simulink model "Task7"  (R2023b)
settings: Solver=VariableStepAuto  StartTime=0.0  StopTime=1800  RelTol=1e-3
InitFcn:
  | run("Linear_Model.m")
values from neighbouring files (symbols this model uses):
  A_Lat = [Yv   Yp+w0   Yr-u0         gravity*cos(theta0)     0 ... (first row only)    [Linear_Model.m]
  A_Long = [Xu                    Xw                        -w0                            -gravity*cos(theta0) ... (first row only)    [Linear_Model.m]
  B_Lat = [Yda          Ydr ... (first row only)    [Linear_Model.m]
  B_Long = [Xde                         Xdth ... (first row only)    [Linear_Model.m]
  C_Lat = eye(5)    [Linear_Model.m]
  C_Long = eye(4)    [Linear_Model.m]
  D_Lat = zeros(5,2)    [Linear_Model.m]
  D_Long = zeros(4,2)    [Linear_Model.m]
  F_gravity_0 = mass*gravity*[sin(states_0(8)) ... (first row only)    [Data_edit.m]
  gravity = Airplane_data(52)    [Data_edit.m]
  Ixx = Airplane_data(53)    [Data_edit.m]
  Iyy = Airplane_data(54)    [Data_edit.m]
  Izz = Airplane_data(55)    [Data_edit.m]
  M0 = [0;0;0]    [Data_edit.m]
  mass = Airplane_data(51)    [Data_edit.m]
  Matrix_controls = [ 0             Xde             Xdth            0 ... (first row only)    [Data_edit.m]
  Matrix_states = [Xu   0   Xw  0   0   0   0 ... (first row only)    [Data_edit.m]
  p0 = states_0(4)    [Data_edit.m]
  phi0 = states_0(7)    [Data_edit.m]
  psi0 = states_0(9)    [Data_edit.m]
  q0 = states_0(5)    [Data_edit.m]
  r0 = states_0(6)    [Data_edit.m]
  states_0 = Airplane_data(4:15)    [Data_edit.m]
  theta0 = states_0(8)    [Data_edit.m]
  u0 = states_0(1)    [Data_edit.m]
  v0 = states_0(2)    [Data_edit.m]
  w0 = states_0(3)    [Data_edit.m]
undefined symbols (not defined in the file or in its folder): Earth, sigbuilder_block, WGS84
libraries: simulink_extras x35, cstblocks x17, slpidlib x12, aerolibasang x2, aerolibfltsims x2, shared6dof x1, dspsigops x1, aerolibtransform2 x1
(part 1 of 2)
settings Model: Creator=saifg  LastModifiedBy=saifg

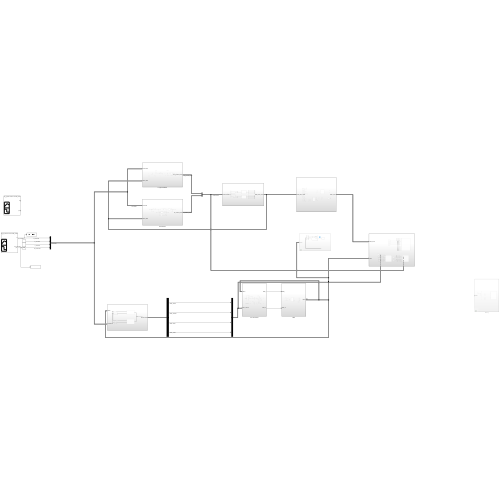
[thumbnail: Simulink's stored preview of the top-level diagram]
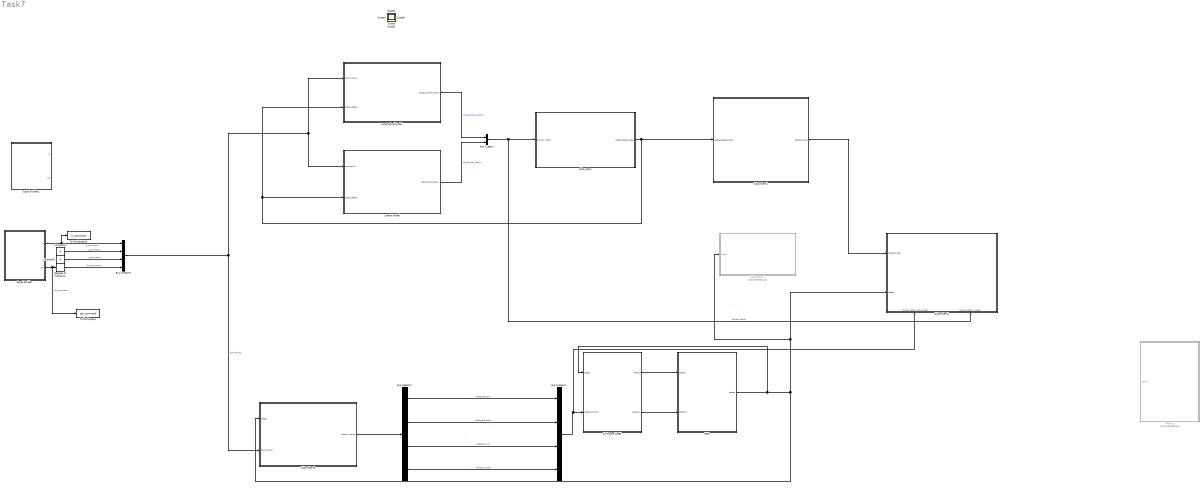
== system Task7 ==
  Air Frame Model : Subsystem
  Bus Creator : BusCreator  Inputs=2
  Bus Creator4 : BusCreator  Inputs=4
  Bus Creator5 : BusCreator  Inputs=4
  Bus Selector : BusSelector  OutputSignals=Lat_Control_Action.delta_aileron,Long_Control_Action.delta_elevator,Long_Control_Action.delta_thrust,Lat_Control_Action.delta_ruuder
  Constant4 : Constant  Value=0
  Constant5 : Constant  Value=0
  Degrees to Radians2 : simulink_extras/Transformations/Degrees to Radians
  "Lateral Model " : Subsystem
  Longitudinal Model : Subsystem
  Plotting : Subsystem  Commented=on
  RBD : Subsystem
  Signal Builder : Subsystem  Tag=STV Subsys  LoadFcn=sigbuilder_block('load');  StartFcn=sigbuilder_block('start');  StopFcn=sigbuilder_block('stop');  ClipboardFcn=sigbuilder_block('clipboard');  mask(Sigbuilder block){tuvar=[0:10]}
      mask help: Simulink:masks:SigbuilderBlock_MD
      mask init:
      | if ~strcmp(get_param(bdroot(gcbh),'SimulationStatus'),'stopped') tuvar = sigbuilder_block('maskInit'); end
      settings: CopyFcn=sigbuilder_block('copy');  DeleteFcn=sigbuilder_block('delete');  ModelCloseFcn=sigbuilder_block('modelClose');  PreSaveFcn=sigbuilder_block('preSave');  PauseFcn=sigbuilder_block('pause');  ContinueFcn=sigbuilder_block('continue');  NameChangeFcn=sigbuilder_block('namechange');  OpenFcn=sigbuilder_block('open',[5.4 36 1141.2 516.6 ]);  CloseFcn=sigbuilder_block('close');
      mask Display: plot(0, 0, 100, 100,[2, 2, 32, 32, 2], [68, 8, 8, 68, 68],[32, 2], [38, 38], [32, 19, 2],[53, 60, 44], [32, 17, 17, 2],[16, 16, 31, 31]);txt = getActiveGroup(gcbh);text(2, 100, txt,'verticalAlignment', 'top');
  Signal Builder1 : Subsystem  Tag=STV Subsys  LoadFcn=sigbuilder_block('load');  StartFcn=sigbuilder_block('start');  StopFcn=sigbuilder_block('stop');  ClipboardFcn=sigbuilder_block('clipboard');  mask(Sigbuilder block){tuvar=[0:10]}
      mask help: Simulink:masks:SigbuilderBlock_MD
      mask init:
      | if ~strcmp(get_param(bdroot(gcbh),'SimulationStatus'),'stopped') tuvar = sigbuilder_block('maskInit'); end
      settings: CopyFcn=sigbuilder_block('copy');  DeleteFcn=sigbuilder_block('delete');  ModelCloseFcn=sigbuilder_block('modelClose');  PreSaveFcn=sigbuilder_block('preSave');  PauseFcn=sigbuilder_block('pause');  ContinueFcn=sigbuilder_block('continue');  NameChangeFcn=sigbuilder_block('namechange');  OpenFcn=sigbuilder_block('open',[5.4 36 1141.2 516.6 ]);  CloseFcn=sigbuilder_block('close');
      mask Display: plot(0, 0, 100, 100,[2, 2, 32, 32, 2], [68, 8, 8, 68, 68],[32, 2], [38, 38], [32, 19, 2],[53, 60, 44], [32, 17, 17, 2],[16, 16, 31, 31]);txt = getActiveGroup(gcbh);text(2, 100, txt,'verticalAlignment', 'top');
  Subsystem : Subsystem
  Subsystem1 : Subsystem
  Subsystem2 : Subsystem
      settings: PortSchema="{\"entries\":[{\"content\":{\"sides\":[{\"content\":{\"connectorIds\":[\"In1\",\"In2\"]},\"type\":\"ConnectorPlacement.EquallySpacedRectSide\",\"uuid\":\"ba0f1933-2a67-495f-a755-837ae570be10\"},{\"content\":{\"side\":\"RIGHT\"},\"type\":\"ConnectorPlacement.EquallySpacedRectSide\",\"uuid\":\"3de798a5-8bce-4885-8633-4329ea784db0\"},{\"content\":{\"side\":\"TOP\"},\"type\":\"ConnectorPlacement.EquallySpacedRectSide\",\"uuid\":\"6ce253ea-975e-40d2-945b-e7cccea3a524\"},{\"content\":{\"connectorIds\":[\"In3\",\"In4\"],\"side\":\"BOTTOM\"},\"type\":\"ConnectorPlacement.EquallySpacedRectSide\",\"uuid\":\"4e7a2a38-3005-49de-8745-c2ef2fbabb58\"}]},\"type\":\"ConnectorPlacement.EquallySpacedConnector\",\"uuid\":\"bc25b1a9-6a92-4f96-820d-23b739a2dded\"}],\"packageUris\":[\"http://schema.mathworks.com/mf0/Connector/R2020b\"],\"version\":\"1.0\"}"
  Subsystem3 : Subsystem
  Subsystem4 : Subsystem  Commented=on
  To Workspace : ToWorkspace  VariableName=psi_command  SampleTime=-1
  To Workspace1 : ToWorkspace  VariableName=H_Command  SampleTime=-1
  Scope{,1..4} (5 alike) : Scope
  wires:
  "Lateral Model "/1(Lat_control_action) -> Bus Creator/2  "Lat_Control_Action"
  Longitudinal Model/1(Long_Control_action) -> Bus Creator/1  "Long_Control_Action"
  Bus Creator/1 -> Subsystem2/4(Conrol Action  Linear), Subsystem/1(Control Action)  "Control Action"
  Subsystem/1(delta_sates_Linear) -> Subsystem1/1(delta_sates_Linear), Longitudinal Model/2(delta_states), "Lateral Model "/2(delta_states)
  Bus Creator5/1 -> Subsystem3/2(Commands), Longitudinal Model/1(Commands), "Lateral Model "/1(command)  "Commands"
  Subsystem1/1(states_linear) -> Subsystem2/1(states_linear)
  Bus Creator4/1 -> Subsystem2/3(Conrol Action Non Linear), Air Frame Model/2(delta_controls)
  RBD/1(states) -> Air Frame Model/1(states), Subsystem4/1(States), Subsystem2/2(states), Subsystem3/1(states)
  Air Frame Model/2(delta_m) -> RBD/2(delta_M)
  Air Frame Model/1(delta_f) -> RBD/1(delta_f)
  Constant5/1 -> Bus Creator5/3  "r_command"
  Constant4/1 -> Bus Creator5/2  "u_command"
  Degrees to Radians2/1 -> Bus Creator5/4  "Psi_command"
  Subsystem3/1(Control Action) -> Bus Selector/1
  Bus Selector/2 -> Bus Creator4/2  "<delta_elevator>"
  Bus Selector/3 -> Bus Creator4/3  "<delta_thrust>"
  Bus Selector/1 -> Bus Creator4/1  "<delta_aileron>"
  Bus Selector/4 -> Bus Creator4/4  "<delta_ruuder>"
  Signal Builder/2(psi) -> To Workspace/1, Degrees to Radians2/1  "Psi_command"
  Signal Builder/1(H) -> To Workspace1/1, Bus Creator5/1  "H_command"

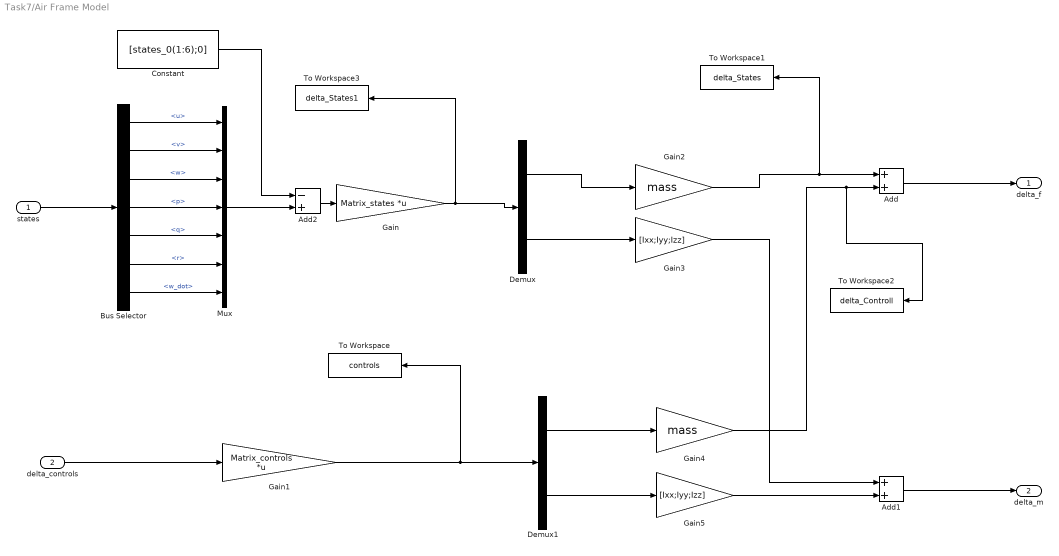
== system Task7/Air Frame Model ==
  states : Inport
  delta_controls : Inport  Port=2
  Add : Sum
  Add1 : Sum
  Add2 : Sum  Inputs=-+
  Bus Selector : BusSelector  OutputSignals=u,v,w,p,q,r,w_dot
  Constant : Constant  Value=[states_0(1:6);0]
  Demux : Demux  Outputs=2
  Demux1 : Demux  Outputs=2
  Gain : Gain  Gain=Matrix_states  Multiplication=Matrix(K*u)
  Gain1 : Gain  Gain=Matrix_controls  Multiplication=Matrix(K*u)
  Gain2 : Gain  Gain=mass
  Gain3 : Gain  Gain=[Ixx;Iyy;Izz]
  Gain4 : Gain  Gain=mass
  Gain5 : Gain  Gain=[Ixx;Iyy;Izz]
  Mux : Mux  Inputs=7
  To Workspace : ToWorkspace  VariableName=controls  SampleTime=-1
  To Workspace1 : ToWorkspace  VariableName=delta_States  SampleTime=-1
  To Workspace2 : ToWorkspace  VariableName=delta_Controll  SampleTime=-1
  To Workspace3 : ToWorkspace  VariableName=delta_States1  SampleTime=-1
  delta_f : Outport
  delta_m : Outport  Port=2
  wires:
  Gain/1 -> To Workspace3/1, Demux/1
  Demux/1 -> Gain2/1
  Demux/2 -> Gain3/1
  Demux1/2 -> Gain5/1
  Demux1/1 -> Gain4/1
  Gain1/1 -> To Workspace/1, Demux1/1
  Gain2/1 -> To Workspace1/1, Add/1
  Gain4/1 -> To Workspace2/1, Add/2
  Gain5/1 -> Add1/2
  Gain3/1 -> Add1/1
  Add/1 -> delta_f/1
  Add1/1 -> delta_m/1
  states/1 -> Bus Selector/1
  Bus Selector/1 -> Mux/1  "<u>"
  Bus Selector/2 -> Mux/2  "<v>"
  Bus Selector/3 -> Mux/3  "<w>"
  Bus Selector/4 -> Mux/4  "<p>"
  Bus Selector/5 -> Mux/5  "<q>"
  Bus Selector/6 -> Mux/6  "<r>"
  Bus Selector/7 -> Mux/7  "<w_dot>"
  Add2/1 -> Gain/1
  Mux/1 -> Add2/2
  Constant/1 -> Add2/1
  delta_controls/1 -> Gain1/1

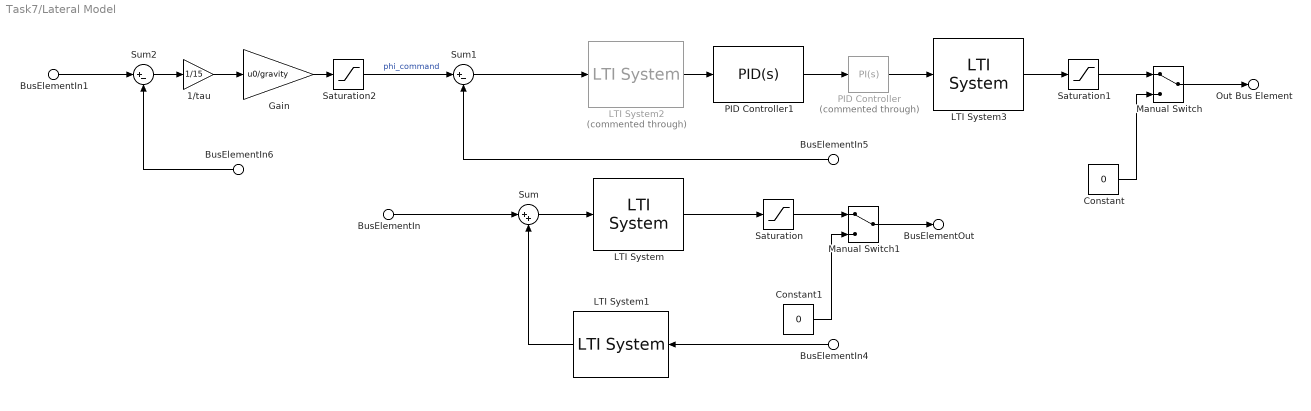
== system Task7/Lateral Model  ==
  BusElementIn : Inport  PortName=command  Element=r_command
  BusElementIn1 : Inport  PortName=command  Element=Psi_command
  BusElementIn4 : Inport  Port=2  PortName=delta_states  Element=delta_r
  BusElementIn5 : Inport  Port=2  PortName=delta_states  Element=delta_phi
  BusElementIn6 : Inport  Port=2  PortName=delta_states  Element=delta_psi
  1/tau : Gain  Gain=1/15
  Constant : Constant  Value=0
  Constant1 : Constant  Value=0
  Gain : Gain  Gain=u0/gravity
  LTI System : cstblocks/LTI System  sys=servo  IC=[]  PadeOrder=0
  LTI System1 : cstblocks/LTI System  sys=HPF_Washout  IC=[]  PadeOrder=0
  LTI System2 : cstblocks/LTI System  Commented=through  sys=Roll_Comp  IC=[]  PadeOrder=0
  LTI System3 : cstblocks/LTI System  sys=servo  IC=[]  PadeOrder=0
  Manual Switch : ManualSwitch
  Manual Switch1 : ManualSwitch
  PID Controller : slpidlib/PID Controller  Commented=through  Controller=PI  Form=Parallel  TimeDomain=Continuous-time  UseExternalTs=off  SampleTime=-1  IntegratorMethod=Forward Euler  FilterMethod=Forward Euler  ControllerParametersSource=internal  P=1.6  I=.0254  UseKiTs=off  D=0  N=100  UseFilter=on  TunerSelectOption=Transfer Function Based (PID Tuner App)  InitialConditionSource=internal  InitialConditionForIntegrator=0  InitialConditionForFilter=0  DifferentiatorICPrevScaledInput=0  ExternalReset=none  TrackingMode=off  Kt=1  LimitOutput=off  SatLimitsSource=internal  UpperSaturationLimit=inf  LowerSaturationLimit=-inf  LinearizeAsGain=on  AntiWindupMode=none  Kb=1  LimitIntegrator=off  UpperIntegratorSaturationLimit=inf  LowerIntegratorSaturationLimit=-inf  POutMin=[]  POutMax=[]  IOutMin=[]  IOutMax=[]  DOutMin=[]  DOutMax=[]  NOutMin=[]  NOutMax=[]  SumOutMin=[]  SumOutMax=[]  SaturationOutMin=[]  SaturationOutMax=[]  PParamMin=[]  PParamMax=[]  IParamMin=[]  IParamMax=[]  DParamMin=[]  DParamMax=[]  NParamMin=[]  NParamMax=[]  KbParamMin=[]  KbParamMax=[]  KtParamMin=[]  KtParamMax=[]  KbOutMin=[]  KbOutMax=[]  KtOutMin=[]  KtOutMax=[]  IntegratorOutMin=[]  IntegratorOutMax=[]  FilterOutMin=[]  FilterOutMax=[]  SumI1OutMin=[]  SumI1OutMax=[]  SumI2OutMin=[]  SumI2OutMax=[]  SumI3OutMin=[]  SumI3OutMax=[]  SumI4OutMin=[]  SumI4OutMax=[]  SumDOutMin=[]  SumDOutMax=[]  DifferentiatorOutMin=[]  DifferentiatorOutMax=[]  FilterDiffOutCoefMin=[]  FilterDiffOutCoefMax=[]  ReciprocalOutMin=[]  ReciprocalOutMax=[]  SumDenOutMin=[]  SumDenOutMax=[]  SumNumOutMin=[]  SumNumOutMax=[]  DivideOutMin=[]  DivideOutMax=[]  UdiffTsProdOutMin=[]  UdiffTsProdOutMax=[]  NTsProdOutMin=[]  NTsProdOutMax=[]  UintegralTsProdOutMin=[]  UintegralTsProdOutMax=[]  UngainTsProdOutMin=[]  UngainTsProdOutMax=[]  ClampingZeroOutDataTypeStr=Inherit: Inherit via back propagation  ClampingZeroOutMin=[]  ClampingZeroOutMax=[]  FilterDenConstantOutDataTypeStr=Inherit: Inherit via back propagation  FilterDenConstantOutMin=[]  FilterDenConstantOutMax=[]  PCopyOutDataTypeStr=Inherit: Inherit via back propagation  PCopyOutMin=[]  PCopyOutMax=[]  NCopyOutDataTypeStr=Inherit: Inherit via back propagation  NCopyOutMin=[]  NCopyOutMax=[]  IntegratorContinuousStateAttributes=''  IntegratorStateMustResolveToSignalObject=off  IntegratorRTWStateStorageClass=Auto  FilterContinuousStateAttributes=''  FilterStateMustResolveToSignalObject=off  FilterRTWStateStorageClass=Auto  ParallelPVariant=InternalParameters  IdealPVariant=Disabled  IVariant=InternalParameters  DVariant=Disabled  IntegratorVariant=Continuous  SatVariant=Disabled  AWVariant=Passthrough  PCopyVariant=Disabled  TRVariant=Disabled  FdbkBlocksVariant=Forward  IdealPFdbkVariant=Disabled  SatFdbkVariant=Disabled  DerivativeFilterVariant=Disabled  NVariant=Disabled  NCopyVariant=Disabled_SignalSpec  FilterICVariant=Disabled  IntegratorICVariant=InternalICs  ExternalResetVariant=Disabled  TRSumVariant=Passthrough  SumFdbkVariant=Disabled  SumVariant=Sum_PI  TsampFilterVariant=InternalTs  TsampNgainVariant=Passthrough  TsampIntegralVariant=Disabled_SignalSpec  ExternalSaturationOutDataTypeStr=Inherit: Same as second input
  PID Controller1 : slpidlib/PID Controller  Controller=PID  Form=Parallel  TimeDomain=Continuous-time  UseExternalTs=off  SampleTime=-1  IntegratorMethod=Forward Euler  FilterMethod=Forward Euler  ControllerParametersSource=internal  P=3.4  I=0.05  UseKiTs=off  D=0.85  N=100  UseFilter=on  TunerSelectOption=Transfer Function Based (PID Tuner App)  InitialConditionSource=internal  InitialConditionForIntegrator=0  InitialConditionForFilter=0  DifferentiatorICPrevScaledInput=0  ExternalReset=none  TrackingMode=off  Kt=1  LimitOutput=off  SatLimitsSource=internal  UpperSaturationLimit=inf  LowerSaturationLimit=-inf  LinearizeAsGain=on  AntiWindupMode=none  Kb=1  LimitIntegrator=off  UpperIntegratorSaturationLimit=inf  LowerIntegratorSaturationLimit=-inf  POutMin=[]  POutMax=[]  IOutMin=[]  IOutMax=[]  DOutMin=[]  DOutMax=[]  NOutMin=[]  NOutMax=[]  SumOutMin=[]  SumOutMax=[]  SaturationOutMin=[]  SaturationOutMax=[]  PParamMin=[]  PParamMax=[]  IParamMin=[]  IParamMax=[]  DParamMin=[]  DParamMax=[]  NParamMin=[]  NParamMax=[]  KbParamMin=[]  KbParamMax=[]  KtParamMin=[]  KtParamMax=[]  KbOutMin=[]  KbOutMax=[]  KtOutMin=[]  KtOutMax=[]  IntegratorOutMin=[]  IntegratorOutMax=[]  FilterOutMin=[]  FilterOutMax=[]  SumI1OutMin=[]  SumI1OutMax=[]  SumI2OutMin=[]  SumI2OutMax=[]  SumI3OutMin=[]  SumI3OutMax=[]  SumI4OutMin=[]  SumI4OutMax=[]  SumDOutMin=[]  SumDOutMax=[]  DifferentiatorOutMin=[]  DifferentiatorOutMax=[]  FilterDiffOutCoefMin=[]  FilterDiffOutCoefMax=[]  ReciprocalOutMin=[]  ReciprocalOutMax=[]  SumDenOutMin=[]  SumDenOutMax=[]  SumNumOutMin=[]  SumNumOutMax=[]  DivideOutMin=[]  DivideOutMax=[]  UdiffTsProdOutMin=[]  UdiffTsProdOutMax=[]  NTsProdOutMin=[]  NTsProdOutMax=[]  UintegralTsProdOutMin=[]  UintegralTsProdOutMax=[]  UngainTsProdOutMin=[]  UngainTsProdOutMax=[]  ClampingZeroOutDataTypeStr=Inherit: Inherit via back propagation  ClampingZeroOutMin=[]  ClampingZeroOutMax=[]  FilterDenConstantOutDataTypeStr=Inherit: Inherit via back propagation  FilterDenConstantOutMin=[]  FilterDenConstantOutMax=[]  PCopyOutDataTypeStr=Inherit: Inherit via back propagation  PCopyOutMin=[]  PCopyOutMax=[]  NCopyOutDataTypeStr=Inherit: Inherit via back propagation  NCopyOutMin=[]  NCopyOutMax=[]  IntegratorContinuousStateAttributes=''  IntegratorStateMustResolveToSignalObject=off  IntegratorRTWStateStorageClass=Auto  FilterContinuousStateAttributes=''  FilterStateMustResolveToSignalObject=off  FilterRTWStateStorageClass=Auto  ParallelPVariant=InternalParameters  IdealPVariant=Disabled  IVariant=InternalParameters  DVariant=InternalParameters  IntegratorVariant=Continuous  SatVariant=Disabled  AWVariant=Passthrough  PCopyVariant=Disabled  TRVariant=Disabled  FdbkBlocksVariant=Forward  IdealPFdbkVariant=Disabled  SatFdbkVariant=Disabled  DerivativeFilterVariant=ContFilter  NVariant=InternalParameters  NCopyVariant=Disabled  FilterICVariant=InternalICsFilter  IntegratorICVariant=InternalICs  ExternalResetVariant=Disabled  TRSumVariant=Passthrough  SumFdbkVariant=Disabled  SumVariant=Sum_PID  TsampFilterVariant=InternalTs  TsampNgainVariant=Passthrough  TsampIntegralVariant=Disabled_SignalSpec  ExternalSaturationOutDataTypeStr=Inherit: Same as second input
  Saturation : Saturate  UpperLimit=deg2rad(30)  LowerLimit=deg2rad(-30)
  Saturation1 : Saturate  UpperLimit=deg2rad(50)  LowerLimit=deg2rad(-50)
  Saturation2 : Saturate  UpperLimit=deg2rad(30)  LowerLimit=deg2rad(-30)
  Sum : Sum  Inputs=|++
  Sum1 : Sum  Inputs=|+-
  Sum2 : Sum  Inputs=|+-
  Out Bus Element : Outport  PortName=Lat_control_action  Element=delta_aileron
  BusElementOut : Outport  PortName=Lat_control_action  Element=delta_ruuder
  wires:
  BusElementIn/1 -> Sum/1
  Sum/1 -> LTI System/1
  LTI System/1 -> Saturation/1
  BusElementIn4/1 -> LTI System1/1
  LTI System1/1 -> Sum/2
  BusElementIn5/1 -> Sum1/2
  Sum1/1 -> LTI System2/1
  LTI System3/1 -> Saturation1/1
  PID Controller/1 -> LTI System3/1
  LTI System2/1 -> PID Controller1/1
  PID Controller1/1 -> PID Controller/1
  BusElementIn6/1 -> Sum2/2
  Gain/1 -> Saturation2/1
  Sum2/1 -> 1/tau/1
  1/tau/1 -> Gain/1
  Saturation2/1 -> Sum1/1  "phi_command"
  BusElementIn1/1 -> Sum2/1
  Saturation1/1 -> Manual Switch/1
  Manual Switch/1 -> Out Bus Element/1
  Constant/1 -> Manual Switch/2
  Constant1/1 -> Manual Switch1/2
  Saturation/1 -> Manual Switch1/1
  Manual Switch1/1 -> BusElementOut/1

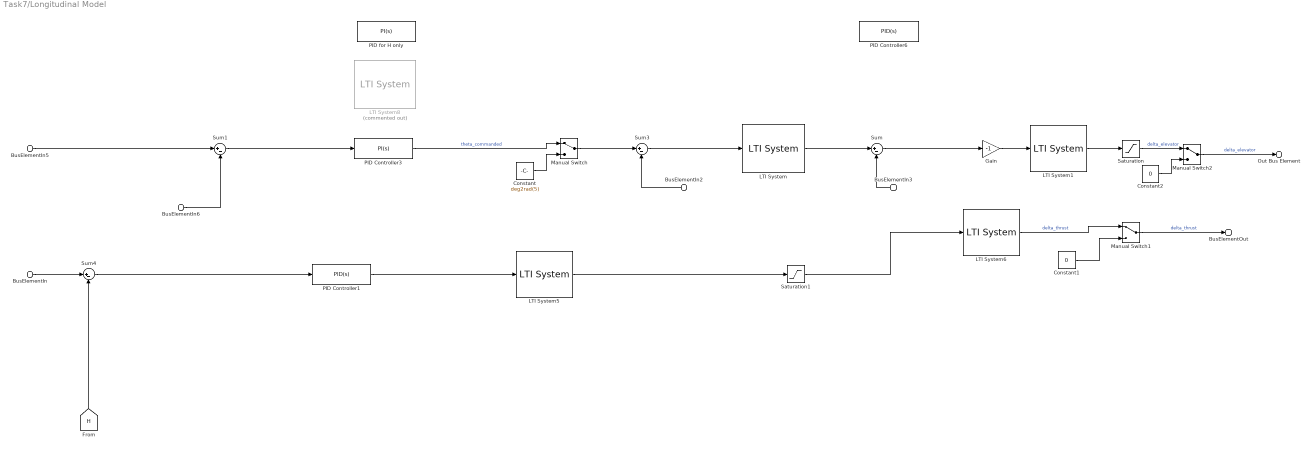
== system Task7/Longitudinal Model ==
  BusElementIn5 : Inport  PortName=Commands  Element=u_command
  BusElementIn : Inport  PortName=Commands  Element=H_command
  BusElementIn6 : Inport  Port=2  PortName=delta_states  Element=delta_u
  BusElementIn2 : Inport  Port=2  PortName=delta_states  Element=delta_theta
  BusElementIn3 : Inport  Port=2  PortName=delta_states  Element=delta_q
  Constant : Constant  Value=deg2rad(5)
  Constant1 : Constant  Value=0
  Constant2 : Constant  Value=0
  Gain : Gain  Gain=-1
  LTI System : cstblocks/LTI System  sys=PI_Pitch  IC=[]  PadeOrder=0
  LTI System1 : cstblocks/LTI System  sys=servo  IC=[]  PadeOrder=0
  LTI System5 : cstblocks/LTI System  sys=servo  IC=[]  PadeOrder=0
  LTI System6 : cstblocks/LTI System  sys=Engine_Lag  IC=[]  PadeOrder=0
  LTI System8 : cstblocks/LTI System  Commented=on  sys=PI_U_theta  IC=[]  PadeOrder=0
  Manual Switch : ManualSwitch
  Manual Switch1 : ManualSwitch
  Manual Switch2 : ManualSwitch
  PID Controller1 : slpidlib/PID Controller  Controller=PID  Form=Parallel  TimeDomain=Continuous-time  UseExternalTs=off  SampleTime=-1  IntegratorMethod=Forward Euler  FilterMethod=Forward Euler  ControllerParametersSource=internal  P=5000  I=.75  UseKiTs=off  D=30000  N=100  UseFilter=on  TunerSelectOption=Transfer Function Based (PID Tuner App)  InitialConditionSource=internal  InitialConditionForIntegrator=0  InitialConditionForFilter=0  DifferentiatorICPrevScaledInput=0  ExternalReset=none  TrackingMode=off  Kt=1  LimitOutput=off  SatLimitsSource=internal  UpperSaturationLimit=inf  LowerSaturationLimit=-inf  LinearizeAsGain=on  AntiWindupMode=none  Kb=1  LimitIntegrator=off  UpperIntegratorSaturationLimit=inf  LowerIntegratorSaturationLimit=-inf  POutMin=[]  POutMax=[]  IOutMin=[]  IOutMax=[]  DOutMin=[]  DOutMax=[]  NOutMin=[]  NOutMax=[]  SumOutMin=[]  SumOutMax=[]  SaturationOutMin=[]  SaturationOutMax=[]  PParamMin=[]  PParamMax=[]  IParamMin=[]  IParamMax=[]  DParamMin=[]  DParamMax=[]  NParamMin=[]  NParamMax=[]  KbParamMin=[]  KbParamMax=[]  KtParamMin=[]  KtParamMax=[]  KbOutMin=[]  KbOutMax=[]  KtOutMin=[]  KtOutMax=[]  IntegratorOutMin=[]  IntegratorOutMax=[]  FilterOutMin=[]  FilterOutMax=[]  SumI1OutMin=[]  SumI1OutMax=[]  SumI2OutMin=[]  SumI2OutMax=[]  SumI3OutMin=[]  SumI3OutMax=[]  SumI4OutMin=[]  SumI4OutMax=[]  SumDOutMin=[]  SumDOutMax=[]  DifferentiatorOutMin=[]  DifferentiatorOutMax=[]  FilterDiffOutCoefMin=[]  FilterDiffOutCoefMax=[]  ReciprocalOutMin=[]  ReciprocalOutMax=[]  SumDenOutMin=[]  SumDenOutMax=[]  SumNumOutMin=[]  SumNumOutMax=[]  DivideOutMin=[]  DivideOutMax=[]  UdiffTsProdOutMin=[]  UdiffTsProdOutMax=[]  NTsProdOutMin=[]  NTsProdOutMax=[]  UintegralTsProdOutMin=[]  UintegralTsProdOutMax=[]  UngainTsProdOutMin=[]  UngainTsProdOutMax=[]  ClampingZeroOutDataTypeStr=Inherit: Inherit via back propagation  ClampingZeroOutMin=[]  ClampingZeroOutMax=[]  FilterDenConstantOutDataTypeStr=Inherit: Inherit via back propagation  FilterDenConstantOutMin=[]  FilterDenConstantOutMax=[]  PCopyOutDataTypeStr=Inherit: Inherit via back propagation  PCopyOutMin=[]  PCopyOutMax=[]  NCopyOutDataTypeStr=Inherit: Inherit via back propagation  NCopyOutMin=[]  NCopyOutMax=[]  IntegratorContinuousStateAttributes=''  IntegratorStateMustResolveToSignalObject=off  IntegratorRTWStateStorageClass=Auto  FilterContinuousStateAttributes=''  FilterStateMustResolveToSignalObject=off  FilterRTWStateStorageClass=Auto  ParallelPVariant=InternalParameters  IdealPVariant=Disabled  IVariant=InternalParameters  DVariant=InternalParameters  IntegratorVariant=Continuous  SatVariant=Disabled  AWVariant=Passthrough  PCopyVariant=Disabled  TRVariant=Disabled  FdbkBlocksVariant=Forward  IdealPFdbkVariant=Disabled  SatFdbkVariant=Disabled  DerivativeFilterVariant=ContFilter  NVariant=InternalParameters  NCopyVariant=Disabled  FilterICVariant=InternalICsFilter  IntegratorICVariant=InternalICs  ExternalResetVariant=Disabled  TRSumVariant=Passthrough  SumFdbkVariant=Disabled  SumVariant=Sum_PID  TsampFilterVariant=InternalTs  TsampNgainVariant=Passthrough  TsampIntegralVariant=Disabled_SignalSpec  ExternalSaturationOutDataTypeStr=Inherit: Same as second input
  PID Controller3 : slpidlib/PID Controller  Controller=PI  Form=Parallel  TimeDomain=Continuous-time  UseExternalTs=off  SampleTime=-1  IntegratorMethod=Forward Euler  FilterMethod=Forward Euler  ControllerParametersSource=internal  P=-0.0029780732187298  I=-6.00662195955179e-05  UseKiTs=off  D=-0.0901078465434796  N=4.30153629977803  UseFilter=on  TunerSelectOption=Transfer Function Based (PID Tuner App)  InitialConditionSource=internal  InitialConditionForIntegrator=0  InitialConditionForFilter=0  DifferentiatorICPrevScaledInput=0  ExternalReset=none  TrackingMode=off  Kt=1  LimitOutput=off  SatLimitsSource=internal  UpperSaturationLimit=inf  LowerSaturationLimit=-inf  LinearizeAsGain=on  AntiWindupMode=none  Kb=1  LimitIntegrator=off  UpperIntegratorSaturationLimit=inf  LowerIntegratorSaturationLimit=-inf  POutMin=[]  POutMax=[]  IOutMin=[]  IOutMax=[]  DOutMin=[]  DOutMax=[]  NOutMin=[]  NOutMax=[]  SumOutMin=[]  SumOutMax=[]  SaturationOutMin=[]  SaturationOutMax=[]  PParamMin=[]  PParamMax=[]  IParamMin=[]  IParamMax=[]  DParamMin=[]  DParamMax=[]  NParamMin=[]  NParamMax=[]  KbParamMin=[]  KbParamMax=[]  KtParamMin=[]  KtParamMax=[]  KbOutMin=[]  KbOutMax=[]  KtOutMin=[]  KtOutMax=[]  IntegratorOutMin=[]  IntegratorOutMax=[]  FilterOutMin=[]  FilterOutMax=[]  SumI1OutMin=[]  SumI1OutMax=[]  SumI2OutMin=[]  SumI2OutMax=[]  SumI3OutMin=[]  SumI3OutMax=[]  SumI4OutMin=[]  SumI4OutMax=[]  SumDOutMin=[]  SumDOutMax=[]  DifferentiatorOutMin=[]  DifferentiatorOutMax=[]  FilterDiffOutCoefMin=[]  FilterDiffOutCoefMax=[]  ReciprocalOutMin=[]  ReciprocalOutMax=[]  SumDenOutMin=[]  SumDenOutMax=[]  SumNumOutMin=[]  SumNumOutMax=[]  DivideOutMin=[]  DivideOutMax=[]  UdiffTsProdOutMin=[]  UdiffTsProdOutMax=[]  NTsProdOutMin=[]  NTsProdOutMax=[]  UintegralTsProdOutMin=[]  UintegralTsProdOutMax=[]  UngainTsProdOutMin=[]  UngainTsProdOutMax=[]  ClampingZeroOutDataTypeStr=Inherit: Inherit via back propagation  ClampingZeroOutMin=[]  ClampingZeroOutMax=[]  FilterDenConstantOutDataTypeStr=Inherit: Inherit via back propagation  FilterDenConstantOutMin=[]  FilterDenConstantOutMax=[]  PCopyOutDataTypeStr=Inherit: Inherit via back propagation  PCopyOutMin=[]  PCopyOutMax=[]  NCopyOutDataTypeStr=Inherit: Inherit via back propagation  NCopyOutMin=[]  NCopyOutMax=[]  IntegratorContinuousStateAttributes=''  IntegratorStateMustResolveToSignalObject=off  IntegratorRTWStateStorageClass=Auto  FilterContinuousStateAttributes=''  FilterStateMustResolveToSignalObject=off  FilterRTWStateStorageClass=Auto  ParallelPVariant=InternalParameters  IdealPVariant=Disabled  IVariant=InternalParameters  DVariant=Disabled  IntegratorVariant=Continuous  SatVariant=Disabled  AWVariant=Passthrough  PCopyVariant=Disabled  TRVariant=Disabled  FdbkBlocksVariant=Forward  IdealPFdbkVariant=Disabled  SatFdbkVariant=Disabled  DerivativeFilterVariant=Disabled  NVariant=Disabled  NCopyVariant=Disabled_SignalSpec  FilterICVariant=Disabled  IntegratorICVariant=InternalICs  ExternalResetVariant=Disabled  TRSumVariant=Passthrough  SumFdbkVariant=Disabled  SumVariant=Sum_PI  TsampFilterVariant=InternalTs  TsampNgainVariant=Passthrough  TsampIntegralVariant=Disabled_SignalSpec  ExternalSaturationOutDataTypeStr=Inherit: Same as second input
  PID Controller6 : slpidlib/PID Controller  Controller=PID  Form=Parallel  TimeDomain=Continuous-time  UseExternalTs=off  SampleTime=-1  IntegratorMethod=Forward Euler  FilterMethod=Forward Euler  ControllerParametersSource=internal  P=3.70277868694912  I=0.831149312790549  UseKiTs=off  D=1.48691502004034  N=20.9794311620465  UseFilter=on  TunerSelectOption=Transfer Function Based (PID Tuner App)  InitialConditionSource=internal  InitialConditionForIntegrator=0  InitialConditionForFilter=0  DifferentiatorICPrevScaledInput=0  ExternalReset=none  TrackingMode=off  Kt=1  LimitOutput=off  SatLimitsSource=internal  UpperSaturationLimit=inf  LowerSaturationLimit=-inf  LinearizeAsGain=on  AntiWindupMode=none  Kb=1  LimitIntegrator=off  UpperIntegratorSaturationLimit=inf  LowerIntegratorSaturationLimit=-inf  POutMin=[]  POutMax=[]  IOutMin=[]  IOutMax=[]  DOutMin=[]  DOutMax=[]  NOutMin=[]  NOutMax=[]  SumOutMin=[]  SumOutMax=[]  SaturationOutMin=[]  SaturationOutMax=[]  PParamMin=[]  PParamMax=[]  IParamMin=[]  IParamMax=[]  DParamMin=[]  DParamMax=[]  NParamMin=[]  NParamMax=[]  KbParamMin=[]  KbParamMax=[]  KtParamMin=[]  KtParamMax=[]  KbOutMin=[]  KbOutMax=[]  KtOutMin=[]  KtOutMax=[]  IntegratorOutMin=[]  IntegratorOutMax=[]  FilterOutMin=[]  FilterOutMax=[]  SumI1OutMin=[]  SumI1OutMax=[]  SumI2OutMin=[]  SumI2OutMax=[]  SumI3OutMin=[]  SumI3OutMax=[]  SumI4OutMin=[]  SumI4OutMax=[]  SumDOutMin=[]  SumDOutMax=[]  DifferentiatorOutMin=[]  DifferentiatorOutMax=[]  FilterDiffOutCoefMin=[]  FilterDiffOutCoefMax=[]  ReciprocalOutMin=[]  ReciprocalOutMax=[]  SumDenOutMin=[]  SumDenOutMax=[]  SumNumOutMin=[]  SumNumOutMax=[]  DivideOutMin=[]  DivideOutMax=[]  UdiffTsProdOutMin=[]  UdiffTsProdOutMax=[]  NTsProdOutMin=[]  NTsProdOutMax=[]  UintegralTsProdOutMin=[]  UintegralTsProdOutMax=[]  UngainTsProdOutMin=[]  UngainTsProdOutMax=[]  ClampingZeroOutDataTypeStr=Inherit: Inherit via back propagation  ClampingZeroOutMin=[]  ClampingZeroOutMax=[]  FilterDenConstantOutDataTypeStr=Inherit: Inherit via back propagation  FilterDenConstantOutMin=[]  FilterDenConstantOutMax=[]  PCopyOutDataTypeStr=Inherit: Inherit via back propagation  PCopyOutMin=[]  PCopyOutMax=[]  NCopyOutDataTypeStr=Inherit: Inherit via back propagation  NCopyOutMin=[]  NCopyOutMax=[]  IntegratorContinuousStateAttributes=''  IntegratorStateMustResolveToSignalObject=off  IntegratorRTWStateStorageClass=Auto  FilterContinuousStateAttributes=''  FilterStateMustResolveToSignalObject=off  FilterRTWStateStorageClass=Auto  ParallelPVariant=InternalParameters  IdealPVariant=Disabled  IVariant=InternalParameters  DVariant=InternalParameters  IntegratorVariant=Continuous  SatVariant=Disabled  AWVariant=Passthrough  PCopyVariant=Disabled  TRVariant=Disabled  FdbkBlocksVariant=Forward  IdealPFdbkVariant=Disabled  SatFdbkVariant=Disabled  DerivativeFilterVariant=ContFilter  NVariant=InternalParameters  NCopyVariant=Disabled  FilterICVariant=InternalICsFilter  IntegratorICVariant=InternalICs  ExternalResetVariant=Disabled  TRSumVariant=Passthrough  SumFdbkVariant=Disabled  SumVariant=Sum_PID  TsampFilterVariant=InternalTs  TsampNgainVariant=Passthrough  TsampIntegralVariant=Disabled_SignalSpec  ExternalSaturationOutDataTypeStr=Inherit: Same as second input
  PID for H only : slpidlib/PID Controller  Controller=PI  Form=Parallel  TimeDomain=Continuous-time  UseExternalTs=off  SampleTime=-1  IntegratorMethod=Forward Euler  FilterMethod=Forward Euler  ControllerParametersSource=internal  P=-0.0037397877140233  I=-5.73690413578542e-05  UseKiTs=off  D=-0.0258377510545885  N=1.36502822030189  UseFilter=on  TunerSelectOption=Transfer Function Based (PID Tuner App)  InitialConditionSource=internal  InitialConditionForIntegrator=0  InitialConditionForFilter=0  DifferentiatorICPrevScaledInput=0  ExternalReset=none  TrackingMode=off  Kt=1  LimitOutput=off  SatLimitsSource=internal  UpperSaturationLimit=inf  LowerSaturationLimit=-inf  LinearizeAsGain=on  AntiWindupMode=none  Kb=1  LimitIntegrator=off  UpperIntegratorSaturationLimit=inf  LowerIntegratorSaturationLimit=-inf  POutMin=[]  POutMax=[]  IOutMin=[]  IOutMax=[]  DOutMin=[]  DOutMax=[]  NOutMin=[]  NOutMax=[]  SumOutMin=[]  SumOutMax=[]  SaturationOutMin=[]  SaturationOutMax=[]  PParamMin=[]  PParamMax=[]  IParamMin=[]  IParamMax=[]  DParamMin=[]  DParamMax=[]  NParamMin=[]  NParamMax=[]  KbParamMin=[]  KbParamMax=[]  KtParamMin=[]  KtParamMax=[]  KbOutMin=[]  KbOutMax=[]  KtOutMin=[]  KtOutMax=[]  IntegratorOutMin=[]  IntegratorOutMax=[]  FilterOutMin=[]  FilterOutMax=[]  SumI1OutMin=[]  SumI1OutMax=[]  SumI2OutMin=[]  SumI2OutMax=[]  SumI3OutMin=[]  SumI3OutMax=[]  SumI4OutMin=[]  SumI4OutMax=[]  SumDOutMin=[]  SumDOutMax=[]  DifferentiatorOutMin=[]  DifferentiatorOutMax=[]  FilterDiffOutCoefMin=[]  FilterDiffOutCoefMax=[]  ReciprocalOutMin=[]  ReciprocalOutMax=[]  SumDenOutMin=[]  SumDenOutMax=[]  SumNumOutMin=[]  SumNumOutMax=[]  DivideOutMin=[]  DivideOutMax=[]  UdiffTsProdOutMin=[]  UdiffTsProdOutMax=[]  NTsProdOutMin=[]  NTsProdOutMax=[]  UintegralTsProdOutMin=[]  UintegralTsProdOutMax=[]  UngainTsProdOutMin=[]  UngainTsProdOutMax=[]  ClampingZeroOutDataTypeStr=Inherit: Inherit via back propagation  ClampingZeroOutMin=[]  ClampingZeroOutMax=[]  FilterDenConstantOutDataTypeStr=Inherit: Inherit via back propagation  FilterDenConstantOutMin=[]  FilterDenConstantOutMax=[]  PCopyOutDataTypeStr=Inherit: Inherit via back propagation  PCopyOutMin=[]  PCopyOutMax=[]  NCopyOutDataTypeStr=Inherit: Inherit via back propagation  NCopyOutMin=[]  NCopyOutMax=[]  IntegratorContinuousStateAttributes=''  IntegratorStateMustResolveToSignalObject=off  IntegratorRTWStateStorageClass=Auto  FilterContinuousStateAttributes=''  FilterStateMustResolveToSignalObject=off  FilterRTWStateStorageClass=Auto  ParallelPVariant=InternalParameters  IdealPVariant=Disabled  IVariant=InternalParameters  DVariant=Disabled  IntegratorVariant=Continuous  SatVariant=Disabled  AWVariant=Passthrough  PCopyVariant=Disabled  TRVariant=Disabled  FdbkBlocksVariant=Forward  IdealPFdbkVariant=Disabled  SatFdbkVariant=Disabled  DerivativeFilterVariant=Disabled  NVariant=Disabled  NCopyVariant=Disabled_SignalSpec  FilterICVariant=Disabled  IntegratorICVariant=InternalICs  ExternalResetVariant=Disabled  TRSumVariant=Passthrough  SumFdbkVariant=Disabled  SumVariant=Sum_PI  TsampFilterVariant=InternalTs  TsampNgainVariant=Passthrough  TsampIntegralVariant=Disabled_SignalSpec  ExternalSaturationOutDataTypeStr=Inherit: Same as second input
  Saturation : Saturate  UpperLimit=deg2rad(25)  LowerLimit=deg2rad(-25)
  Saturation1 : Saturate  UpperLimit=65369  LowerLimit=-269369.84
  Sum{,1,3..4} (4 alike) : Sum  Inputs=|+-
  Out Bus Element : Outport  PortName=Long_Control_action  Element=delta_elevator
  BusElementOut : Outport  PortName=Long_Control_action  Element=delta_thrust
  wires:
  LTI System1/1 -> Saturation/1
  Gain/1 -> LTI System1/1
  Sum/1 -> Gain/1
  LTI System/1 -> Sum/1
  Sum3/1 -> LTI System/1
  BusElementIn6/1 -> Sum1/2
  BusElementIn2/1 -> Sum3/2
  BusElementIn3/1 -> Sum/2
  BusElementIn/1 -> Sum4/1
  LTI System5/1 -> Saturation1/1
  Saturation1/1 -> LTI System6/1
  [H] -> Sum4/2
  Sum4/1 -> PID Controller1/1
  PID Controller1/1 -> LTI System5/1
  Sum1/1 -> PID Controller3/1
  PID Controller3/1 -> Manual Switch/1  "theta_commanded"
  Manual Switch/1 -> Sum3/1
  Constant/1 -> Manual Switch/2
  LTI System6/1 -> Manual Switch1/1  "delta_thrust"
  Manual Switch1/1 -> BusElementOut/1  "delta_thrust"
  Constant1/1 -> Manual Switch1/2
  BusElementIn5/1 -> Sum1/1
  Saturation/1 -> Manual Switch2/1  "delta_elevator"
  Manual Switch2/1 -> Out Bus Element/1  "delta_elevator"
  Constant2/1 -> Manual Switch2/2

== system Task7/Plotting ==
  states : Inport
  Bus Selector : BusSelector  OutputSignals=x,y,z,phi,ceta,psi,u,v,w,p,q,r
  Radians to Degrees{,1..5} (6 alike) : simulink_extras/Transformations/Radians to Degrees
  Scope : Scope  NumInputPorts=12
  To Workspace3 : ToWorkspace  VariableName=states  SampleTime=-1
  wires:
  states/1 -> To Workspace3/1, Bus Selector/1
  Bus Selector/1 -> Scope/1  "<x>"
  Bus Selector/2 -> Scope/2  "<y>"
  Bus Selector/3 -> Scope/3  "<z>"
  Bus Selector/4 -> Radians to Degrees/1  "<phi>"
  Bus Selector/5 -> Radians to Degrees1/1  "<ceta>"
  Bus Selector/6 -> Radians to Degrees2/1  "<psi>"
  Bus Selector/7 -> Scope/7  "<u>"
  Bus Selector/8 -> Scope/8  "<v>"
  Bus Selector/9 -> Scope/9  "<w>"
  Bus Selector/10 -> Radians to Degrees3/1  "<p>"
  Bus Selector/11 -> Radians to Degrees4/1  "<q>"
  Bus Selector/12 -> Radians to Degrees5/1  "<r>"
  Radians to Degrees/1 -> Scope/4  "phi"
  Radians to Degrees1/1 -> Scope/5  "ceta"
  Radians to Degrees2/1 -> Scope/6  "psi"
  Radians to Degrees3/1 -> Scope/10  "p"
  Radians to Degrees4/1 -> Scope/11  "q"
  Radians to Degrees5/1 -> Scope/12  "r"

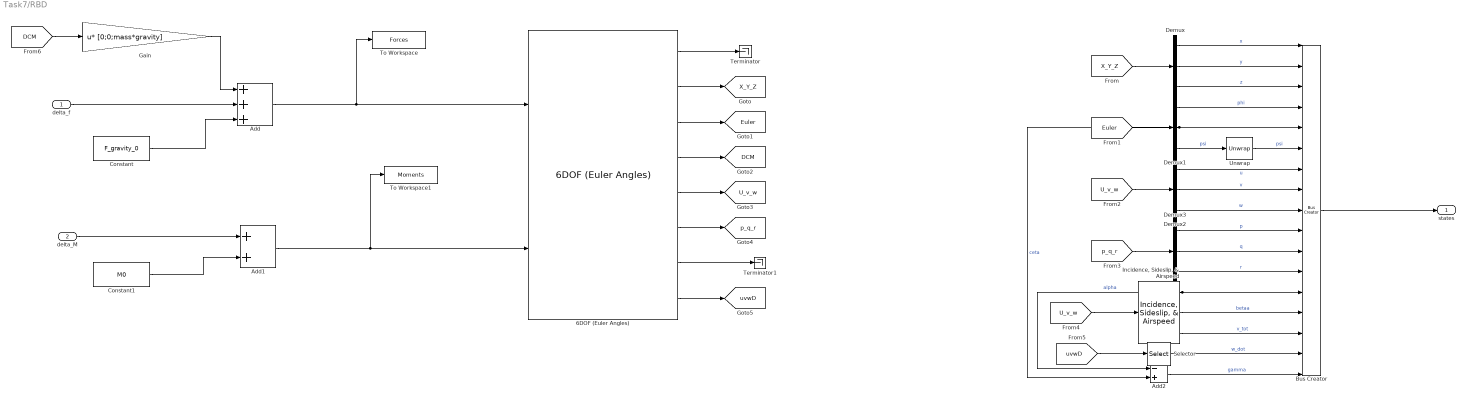
== system Task7/RBD ==
  delta_f : Inport
  delta_M : Inport  Port=2
  6DOF (Euler Angles) : shared6dof/6DOF (Euler Angles)  units=English (Velocity in ft/s)  mtype=Fixed  rep=Euler Angles  xme_0=states_0(10:12)  Vm_0=states_0(1:3)  eul_0=states_0(7:9)  pm_0=states_0(4:6)  mass_0=mass  mass_e=0.5  mass_f=2.0  inertia=I  inertia_e=eye(3)  inertia_f=2*eye(3)  k_quat=1.0  vre_flag=on  abi_flag=off  aMode=0  xme_statename=''  Vm_statename=''  eul_statename=''  quat_statename=''  pm_statename=''  mass_statename=''
  Add : Sum  Inputs=+++
  Add1 : Sum
  Add2 : Sum  Inputs=-+
  Bus Creator : BusCreator  Inputs=17
  Constant : Constant  Value=F_gravity_0
  Constant1 : Constant  Value=M0
  Demux{,1..3} (4 alike) : Demux  Outputs=3
  Gain : Gain  Gain=[0;0;mass*gravity]  Multiplication=Matrix(u*K)
  "Incidence, Sideslip, & Airspeed" : aerolibasang/Incidence, Sideslip, & Airspeed
  Selector : Selector  InputPortWidth=3  IndexOptions=Index vector (dialog)  Indices=[3]  OutputSizes=1
  Terminator : Terminator
  Terminator1 : Terminator
  To Workspace : ToWorkspace  VariableName=Forces  SampleTime=-1
  To Workspace1 : ToWorkspace  VariableName=Moments  SampleTime=-1
  Unwrap : dspsigops/Unwrap  tol=pi  InputProcessing=Columns as channels (frame based)  running=off
  states : Outport
  tag scope: DCM=global, Euler=global, U_v_w=global, X_Y_Z=global, p_q_r=global, uvwD=global
  wires:
  6DOF (Euler Angles)/1 -> Terminator/1
  6DOF (Euler Angles)/2 -> [X_Y_Z]
  6DOF (Euler Angles)/3 -> [Euler]
  6DOF (Euler Angles)/4 -> [DCM]
  6DOF (Euler Angles)/5 -> [U_v_w]
  6DOF (Euler Angles)/6 -> [p_q_r]
  6DOF (Euler Angles)/7 -> Terminator1/1
  6DOF (Euler Angles)/8 -> [uvwD]
  [X_Y_Z] -> Demux/1
  [Euler] -> Demux1/1
  [U_v_w] -> Demux2/1
  [p_q_r] -> Demux3/1
  Demux/1 -> Bus Creator/1  "x"
  Demux/2 -> Bus Creator/2  "y"
  Demux1/1 -> Bus Creator/4  "phi"
  Demux1/3 -> Unwrap/1  "psi"
  Demux2/1 -> Bus Creator/7  "u"
  Demux2/2 -> Bus Creator/8  "v"
  Demux2/3 -> Bus Creator/9  "w"
  Demux3/1 -> Bus Creator/10  "p"
  Demux3/2 -> Bus Creator/11  "q"
  Demux3/3 -> Bus Creator/12  "r"
  [U_v_w] -> "Incidence, Sideslip, & Airspeed"/1
  "Incidence, Sideslip, & Airspeed"/2 -> Bus Creator/14  "betaa"
  "Incidence, Sideslip, & Airspeed"/1 -> Bus Creator/13, Add2/1  "alpha"
  "Incidence, Sideslip, & Airspeed"/3 -> Bus Creator/15  "v_tot"
  [uvwD] -> Selector/1
  Selector/1 -> Bus Creator/16  "w_dot"
  Bus Creator/1 -> states/1
  delta_f/1 -> Add/2
  [DCM] -> Gain/1
  Gain/1 -> Add/1
  Constant/1 -> Add/3
  delta_M/1 -> Add1/1
  Constant1/1 -> Add1/2
  Add1/1 -> To Workspace1/1, 6DOF (Euler Angles)/2
  Unwrap/1 -> Bus Creator/6  "psi"
  Add/1 -> To Workspace/1, 6DOF (Euler Angles)/1
  Demux/3 -> Bus Creator/3  "z"
  Add2/1 -> Bus Creator/17  "gamma"
  Demux1/2 -> Bus Creator/5, Add2/2  "ceta"

== system Task7/Signal Builder ==
  Demux : Demux  Tag=STV Demux  Outputs=2
      settings: DisplayOption=none
  FromWs : FromWorkspace  Tag=STV FromWs  VariableName=tuvar
      SigBuilderData=|
      | common.afterFinalStr = 'Extrapolate'
      | common.sampleTime = 0
      | dataSet.timeRange = [0 2000]
      | dataSet.name = 'log_0_2021-4-14-21-54-39_vehicl'
      | sbobj.Name = 'Signal Builder'
      | sbobj.Groups.Name = 'log_0_2021-4-14-21-54-39_vehicl'
      | sbobj.Groups.Signals(1).Name = 'H'
      | sbobj.Groups.Signals(1).XData = [0 600 1080 1080 1200 1800 2000]
      | sbobj.Groups.Signals(1).YData = [0 10000 10000 10100 10100 0 0]
      | sbobj.Groups.Signals(2).Name = 'psi'
      | sbobj.Groups.Signals(2).XData = [0 720 720 1080 1080 2000]
      | sbobj.Groups.Signals(2).YData = [0 0 360 360 390 390]
      | sbobj.Groups.TimeRange = [0 2000]
  H : Outport  Tag=STV Outport
  psi : Outport  Tag=STV Outport  Port=2
  wires:
  FromWs/1 -> Demux/1
  Demux/1 -> H/1
  Demux/2 -> psi/1

== system Task7/Signal Builder1 ==
  Demux : Demux  Tag=STV Demux  Outputs=2
      settings: DisplayOption=none
  FromWs : FromWorkspace  Tag=STV FromWs  VariableName=tuvar
      SigBuilderData=|
      | common.afterFinalStr = 'Extrapolate'
      | common.sampleTime = 0
      | dataSet.timeRange = [0 2000]
      | dataSet.name = 'log_0_2021-4-14-21-54-39_vehicl'
      | sbobj.Name = 'Signal Builder'
      | sbobj.Groups.Name = 'log_0_2021-4-14-21-54-39_vehicl'
      | sbobj.Groups.Signals(1).Name = 'H'
      | sbobj.Groups.Signals(1).XData = [0 400.002 880.002 880.002 1000.002 1420.002 2000]
      | sbobj.Groups.Signals(1).YData = [0 10000 10000 10100 10100 0 0]
      | sbobj.Groups.Signals(2).Name = 'psi'
      | sbobj.Groups.Signals(2).XData = [0 880.002 880.002 1000.002 1000.002 2000]
      | sbobj.Groups.Signals(2).YData = [0 0 360 360 390 390]
      | sbobj.Groups.TimeRange = [0 2000]
  H : Outport  Tag=STV Outport
  psi : Outport  Tag=STV Outport  Port=2
  wires:
  FromWs/1 -> Demux/1
  Demux/1 -> H/1
  Demux/2 -> psi/1

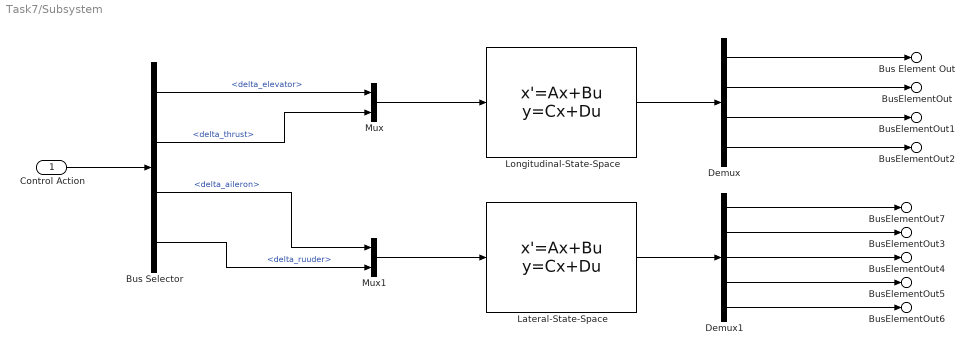
== system Task7/Subsystem ==
  Control Action : Inport
  Bus Selector : BusSelector  OutputSignals=Long_Control_Action.delta_elevator,Long_Control_Action.delta_thrust,Lat_Control_Action.delta_aileron,Lat_Control_Action.delta_ruuder
  Demux : Demux
  Demux1 : Demux  Outputs=5
  Lateral-State-Space : StateSpace  A=A_Lat  B=B_Lat  C=C_Lat  D=D_Lat  InitialCondition=0
  Longitudinal-State-Space : StateSpace  A=A_Long  B=B_Long  C=C_Long  D=D_Long  InitialCondition=0
  Mux : Mux  Inputs=2
  Mux1 : Mux  Inputs=2
  Bus Element Out : Outport  PortName=delta_sates_Linear  Element=delta_u
  BusElementOut : Outport  PortName=delta_sates_Linear  Element=delta_w
  BusElementOut1 : Outport  PortName=delta_sates_Linear  Element=delta_q
  BusElementOut2 : Outport  PortName=delta_sates_Linear  Element=delta_theta
  BusElementOut3 : Outport  PortName=delta_sates_Linear  Element=delta_p
  BusElementOut4 : Outport  PortName=delta_sates_Linear  Element=delta_r
  BusElementOut5 : Outport  PortName=delta_sates_Linear  Element=delta_phi
  BusElementOut6 : Outport  PortName=delta_sates_Linear  Element=delta_psi
  BusElementOut7 : Outport  PortName=delta_sates_Linear  Element=delta_v
  wires:
  Longitudinal-State-Space/1 -> Demux/1
  Mux1/1 -> Lateral-State-Space/1
  Mux/1 -> Longitudinal-State-Space/1
  Lateral-State-Space/1 -> Demux1/1
  Demux1/1 -> BusElementOut7/1
  Demux1/2 -> BusElementOut3/1
  Demux1/3 -> BusElementOut4/1
  Demux1/4 -> BusElementOut5/1
  Demux1/5 -> BusElementOut6/1
  Demux/1 -> Bus Element Out/1
  Demux/2 -> BusElementOut/1
  Demux/3 -> BusElementOut1/1
  Demux/4 -> BusElementOut2/1
  Control Action/1 -> Bus Selector/1
  Bus Selector/1 -> Mux/1  "<delta_elevator>"
  Bus Selector/2 -> Mux/2  "<delta_thrust>"
  Bus Selector/4 -> Mux1/2  "<delta_ruuder>"
  Bus Selector/3 -> Mux1/1  "<delta_aileron>"

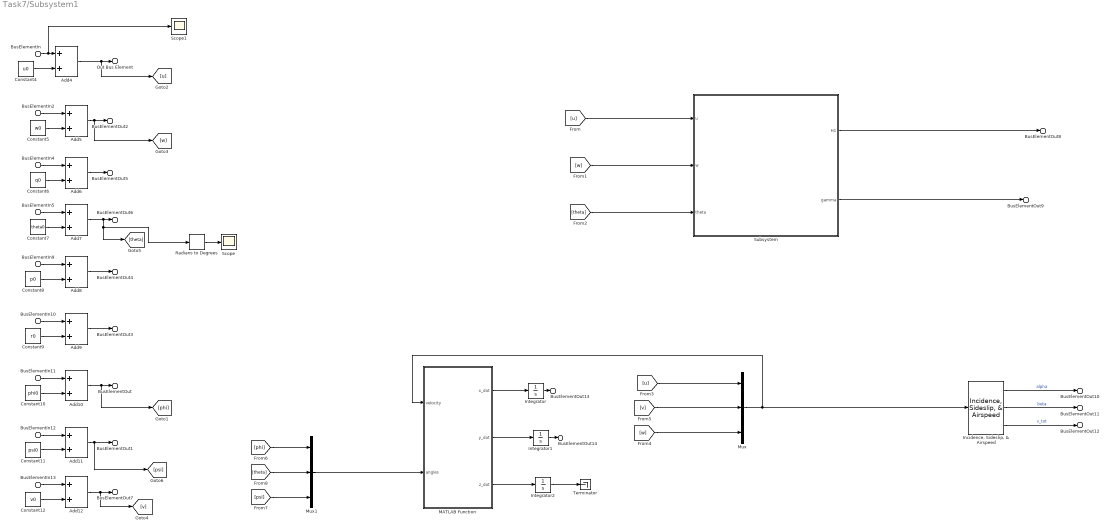
== system Task7/Subsystem1 ==
  BusElementIn : Inport  PortName=delta_sates_Linear  Element=delta_u
  BusElementIn2 : Inport  PortName=delta_sates_Linear  Element=delta_w
  BusElementIn4 : Inport  PortName=delta_sates_Linear  Element=delta_q
  BusElementIn5 : Inport  PortName=delta_sates_Linear  Element=delta_theta
  BusElementIn9 : Inport  PortName=delta_sates_Linear  Element=delta_p
  BusElementIn10 : Inport  PortName=delta_sates_Linear  Element=delta_r
  BusElementIn11 : Inport  PortName=delta_sates_Linear  Element=delta_phi
  BusElementIn12 : Inport  PortName=delta_sates_Linear  Element=delta_psi
  BusElementIn13 : Inport  PortName=delta_sates_Linear  Element=delta_v
  Add{4..12} (9 alike) : Sum
  Constant10 : Constant  Value=phi0
  Constant11 : Constant  Value=psi0
  Constant12 : Constant  Value=v0
  Constant4 : Constant  Value=u0
  Constant5 : Constant  Value=w0
  Constant6 : Constant  Value=q0
  Constant7 : Constant  Value=theta0
  Constant8 : Constant  Value=p0
  Constant9 : Constant  Value=r0
  "Incidence, Sideslip, & Airspeed" : aerolibasang/Incidence, Sideslip, & Airspeed
  Integrator : Integrator
  Integrator1 : Integrator
  Integrator2 : Integrator
  MATLAB Function : MATLAB Function  TreatAsAtomicUnit=on
  Mux : Mux  Inputs=3
  Mux1 : Mux  Inputs=3
  Radians to Degrees : simulink_extras/Transformations/Radians to Degrees
  Scope : Scope
  Scope1 : Scope
  Subsystem : Subsystem
  Terminator : Terminator
  Out Bus Element : Outport  PortName=states_linear  Element=u
  BusElementOut2 : Outport  PortName=states_linear  Element=w
  BusElementOut3 : Outport  PortName=states_linear  Element=r
  BusElementOut4 : Outport  PortName=states_linear  Element=p
  BusElementOut5 : Outport  PortName=states_linear  Element=q
  BusElementOut6 : Outport  PortName=states_linear  Element=theta
  BusElementOut : Outport  PortName=states_linear  Element=phi
  BusElementOut1 : Outport  PortName=states_linear  Element=psi
  BusElementOut7 : Outport  PortName=states_linear  Element=v
  BusElementOut8 : Outport  PortName=states_linear  Element=H
  BusElementOut9 : Outport  PortName=states_linear  Element=gamma(rad)
  BusElementOut10 : Outport  PortName=states_linear  Element=alpha
  BusElementOut11 : Outport  PortName=states_linear  Element=beta
  BusElementOut12 : Outport  PortName=states_linear  Element=v_tot
  BusElementOut13 : Outport  PortName=states_linear  Element=x
  BusElementOut14 : Outport  PortName=states_linear  Element=y
  wires:
  Constant4/1 -> Add4/2
  BusElementIn/1 -> Scope1/1, Add4/1
  Add4/1 -> [u], Out Bus Element/1
  BusElementIn2/1 -> Add5/1
  Constant5/1 -> Add5/2
  Add5/1 -> [w], BusElementOut2/1
  BusElementIn4/1 -> Add6/1
  Constant6/1 -> Add6/2
  BusElementIn5/1 -> Add7/1
  Constant7/1 -> Add7/2
  BusElementIn9/1 -> Add8/1
  Constant8/1 -> Add8/2
  BusElementIn10/1 -> Add9/1
  Constant9/1 -> Add9/2
  BusElementIn11/1 -> Add10/1
  Constant10/1 -> Add10/2
  BusElementIn12/1 -> Add11/1
  Constant11/1 -> Add11/2
  BusElementIn13/1 -> Add12/1
  Constant12/1 -> Add12/2
  Add6/1 -> BusElementOut5/1
  Add8/1 -> BusElementOut4/1
  Add7/1 -> Radians to Degrees/1, [theta], BusElementOut6/1
  Add9/1 -> BusElementOut3/1
  Add10/1 -> [phi], BusElementOut/1
  Add11/1 -> [psi], BusElementOut1/1
  Add12/1 -> [v], BusElementOut7/1
  Subsystem/1(H1) -> BusElementOut8/1
  Subsystem/2(gamma) -> BusElementOut9/1
  [u] -> Subsystem/1(u)
  [theta] -> Subsystem/3(theta)
  [w] -> Subsystem/2(w)
  Mux/1 -> MATLAB Function/1(velocity), "Incidence, Sideslip, & Airspeed"/1
  [u] -> Mux/1
  [w] -> Mux/3
  [v] -> Mux/2
  "Incidence, Sideslip, & Airspeed"/1 -> BusElementOut10/1  "alpha"
  "Incidence, Sideslip, & Airspeed"/2 -> BusElementOut11/1  "beta"
  "Incidence, Sideslip, & Airspeed"/3 -> BusElementOut12/1  "v_tot"
  [phi] -> Mux1/1
  [theta] -> Mux1/2
  [psi] -> Mux1/3
  Mux1/1 -> MATLAB Function/2(angles)
  MATLAB Function/1(x_dot) -> Integrator/1
  MATLAB Function/2(y_dot) -> Integrator1/1
  MATLAB Function/3(z_dot) -> Integrator2/1
  Integrator1/1 -> BusElementOut14/1
  Integrator/1 -> BusElementOut13/1
  Integrator2/1 -> Terminator/1
  Radians to Degrees/1 -> Scope/1
